simulink model "mf14_100"  (R2023b)
(part 2 of 10)

  u80/1 -> Sum158/2
  Sum123/1 -> Stick Input51/1, Controller51/1(Stick Input (in))
  Nz pilot calculation78/1(Pilot g force (g)) -> Pilot G force Scope78/1, Nz Pilot (g)84/1
  Dryden Wind Gust Models64/1(Wg) -> Gain220/1, Gain206/1  "wGust"
  Gain231/1 -> Sum174/1
  Sum177/1 -> Stick Input78/1, Controller78/1(Stick Input (in))
  Sum162/1 -> Stick Input80/1, Controller80/1(Stick Input (in))
  Pilot62/1 -> Sum145/1
  Sum113/1 -> Aircraft Dynamics Model52/3(Rotary Gust qGust (rad/sec))
  Controller77/1(Elevator Command (deg)) -> Actuator Model77/1
  Nz pilot calculation77/1(Pilot g force (g)) -> Pilot G force Scope77/1, Nz Pilot (g)83/1
  Controller70/1(Elevator Command (deg)) -> Actuator Model70/1
  Nz pilot calculation80/1(Pilot g force (g)) -> Pilot G force Scope80/1, Nz Pilot (g)86/1
  Sum104/1 -> Aircraft Dynamics Model96/3(Rotary Gust qGust (rad/sec))
  Gain237/1 -> alpha (rad)84/1, Angle of Attack78/1, Controller78/2(alpha (rad))
  Dryden Wind Gust Models78/2(Qg) -> Gain233/1  "qGust"
  Actuator Model81/1 -> Aircraft Dynamics Model81/1(Elevator Deflection d (deg))
  Dryden Wind Gust Models76/2(Qg) -> Gain267/1  "qGust"
  Gain221/1 -> alpha (rad)71/1, Angle of Attack64/1, Controller64/2(alpha (rad))
  Gain333/1 -> Sum106/2
  Dryden Wind Gust Models59/1(Wg) -> Gain351/1, Gain370/1  "wGust"
  Controller80/1(Elevator Command (deg)) -> Actuator Model80/1
  Gain367/1 -> alpha (rad)51/1, Angle of Attack51/1, Controller51/2(alpha (rad))
  Dryden Wind Gust Models87/1(Wg) -> Gain271/1, Gain310/1  "wGust"
  u56/1 -> Sum105/2
  Sum109/1 -> Stick Input98/1, Controller98/1(Stick Input (in))
  Aircraft Dynamics Model61/2(Pitch Rate q (rad/sec)) -> Nz pilot calculation61/2(q), Controller61/3(q (rad/sec))  "q"
  Dryden Wind Gust Models74/1(Wg) -> Gain238/1, Gain225/1  "wGust"
  Gain309/1 -> alpha (rad)91/1, Angle of Attack86/1, Controller86/2(alpha (rad))
  Nz pilot calculation99/1(Pilot g force (g)) -> Pilot G force Scope99/1, Nz Pilot (g)59/1
  Pilot91/1 -> Sum184/1
  Sum101/1 -> Stick Input50/1, Controller50/1(Stick Input (in))
  Sum138/1 -> Stick Input68/1, Controller68/1(Stick Input (in))
  Actuator Model97/1 -> Aircraft Dynamics Model97/1(Elevator Deflection d (deg))
  Sum157/1 -> Aircraft Dynamics Model74/3(Rotary Gust qGust (rad/sec))
  Controller62/1(Elevator Command (deg)) -> Actuator Model62/1
  Aircraft Dynamics Model75/1(Vertical Velocity w (ft/sec)) -> Gain265/1, Nz pilot calculation75/1(w)  "w"
  Gain287/1 -> Aircraft Dynamics Model93/2(Vertical Gust wGust (ft/sec))
  u91/1 -> Sum193/2
  Nz pilot calculation51/1(Pilot g force (g)) -> Pilot G force Scope51/1, Nz Pilot (g)51/1
  Sum187/1 -> Aircraft Dynamics Model93/3(Rotary Gust qGust (rad/sec))
  Aircraft Dynamics Model76/1(Vertical Velocity w (ft/sec)) -> Gain228/1, Nz pilot calculation76/1(w)  "w"
  u98/1 -> Sum188/2
  Sum199/1 -> Stick Input89/1, Controller89/1(Stick Input (in))
  Gain380/1 -> Sum135/2
  Gain259/1 -> alpha (rad)86/1, Angle of Attack80/1, Controller80/2(alpha (rad))
  Gain318/1 -> Sum108/2
  Dryden Wind Gust Models85/2(Qg) -> Gain270/1  "qGust"
  Gain248/1 -> Sum168/2
  Nz pilot calculation56/1(Pilot g force (g)) -> Pilot G force Scope56/1, Nz Pilot (g)64/1
  Sum128/1 -> Aircraft Dynamics Model54/3(Rotary Gust qGust (rad/sec))
  Dryden Wind Gust Models90/1(Wg) -> Gain297/1, Gain283/1  "wGust"
  Gain250/1 -> Aircraft Dynamics Model75/2(Vertical Gust wGust (ft/sec))
  Gain292/1 -> Sum190/2
  Gain308/1 -> Sum192/1
  Aircraft Dynamics Model85/2(Pitch Rate q (rad/sec)) -> Nz pilot calculation85/2(q), Controller85/3(q (rad/sec))  "q"
  Nz pilot calculation86/1(Pilot g force (g)) -> Pilot G force Scope86/1, Nz Pilot (g)91/1
  Gain307/1 -> alpha (rad)90/1, Angle of Attack85/1, Controller85/2(alpha (rad))
  Sum144/1 -> Stick Input71/1, Controller71/1(Stick Input (in))
  Controller92/1(Elevator Command (deg)) -> Actuator Model92/1
  Gain234/1 -> alpha (rad)83/1, Angle of Attack77/1, Controller77/2(alpha (rad))
  Sum179/1 -> Aircraft Dynamics Model85/3(Rotary Gust qGust (rad/sec))
  u90/1 -> Sum180/2
  Gain270/1 -> Sum179/2
  Gain364/1 -> Aircraft Dynamics Model58/2(Vertical Gust wGust (ft/sec))
  Pilot70/1 -> Sum142/1
  Pilot80/1 -> Sum162/1
  Sum135/1 -> Aircraft Dynamics Model63/3(Rotary Gust qGust (rad/sec))
  Actuator Model71/1 -> Aircraft Dynamics Model71/1(Elevator Deflection d (deg))
  Aircraft Dynamics Model92/2(Pitch Rate q (rad/sec)) -> Nz pilot calculation92/2(q), Controller92/3(q (rad/sec))  "q"
  Sum117/1 -> Aircraft Dynamics Model58/3(Rotary Gust qGust (rad/sec))
  Gain286/1 -> alpha (rad)97/1, Angle of Attack92/1, Controller92/2(alpha (rad))
  Gain360/1 -> Aircraft Dynamics Model53/2(Vertical Gust wGust (ft/sec))
  Gain219/1 -> alpha (rad)70/1, Angle of Attack63/1, Controller63/2(alpha (rad))
  Gain365/1 -> Sum117/2
  u97/1 -> Sum186/2
  Dryden Wind Gust Models86/1(Wg) -> Gain308/1, Gain294/1  "wGust"
  Gain304/1 -> Aircraft Dynamics Model92/2(Vertical Gust wGust (ft/sec))
  Controller79/1(Elevator Command (deg)) -> Actuator Model79/1
  u61/1 -> Sum127/2
  Aircraft Dynamics Model98/1(Vertical Velocity w (ft/sec)) -> Gain322/1, Nz pilot calculation98/1(w)  "w"
  Aircraft Dynamics Model79/2(Pitch Rate q (rad/sec)) -> Nz pilot calculation79/2(q), Controller79/3(q (rad/sec))  "q"
  Aircraft Dynamics Model90/1(Vertical Velocity w (ft/sec)) -> Gain300/1, Nz pilot calculation90/1(w)  "w"
  Aircraft Dynamics Model82/1(Vertical Velocity w (ft/sec)) -> Gain249/1, Nz pilot calculation82/1(w)  "w"
  Controller82/1(Elevator Command (deg)) -> Actuator Model82/1
  Sum196/1 -> Aircraft Dynamics Model88/3(Rotary Gust qGust (rad/sec))
  Actuator Model91/1 -> Aircraft Dynamics Model91/1(Elevator Deflection d (deg))
  u64/1 -> Sum133/2
  Aircraft Dynamics Model93/1(Vertical Velocity w (ft/sec)) -> Gain293/1, Nz pilot calculation93/1(w)  "w"
  Sum185/1 -> Aircraft Dynamics Model92/3(Rotary Gust qGust (rad/sec))
  Gain285/1 -> Sum185/1
  Gain335/1 -> Aircraft Dynamics Model52/2(Vertical Gust wGust (ft/sec))
  u69/1 -> Sum125/2
  Dryden Wind Gust Models84/1(Wg) -> Gain290/1, Gain257/1  "wGust"
  Dryden Wind Gust Models92/2(Qg) -> Gain305/1  "qGust"
  Nz pilot calculation90/1(Pilot g force (g)) -> Pilot G force Scope90/1, Nz Pilot (g)95/1
  u82/1 -> Sum173/2
  Nz pilot calculation92/1(Pilot g force (g)) -> Pilot G force Scope92/1, Nz Pilot (g)97/1
  Nz pilot calculation68/1(Pilot g force (g)) -> Pilot G force Scope68/1, Nz Pilot (g)75/1
  Sum111/1 -> Stick Input99/1, Controller99/1(Stick Input (in))
  Sum147/1 -> Stick Input72/1, Controller72/1(Stick Input (in))
  Dryden Wind Gust Models89/2(Qg) -> Gain277/1  "qGust"
  Dryden Wind Gust Models83/1(Wg) -> Gain251/1, Gain247/1  "wGust"
  Controller67/1(Elevator Command (deg)) -> Actuator Model67/1
  Controller98/1(Elevator Command (deg)) -> Actuator Model98/1
  Gain358/1 -> Sum124/2
  Dryden Wind Gust Models92/1(Wg) -> Gain285/1, Gain304/1  "wGust"
  Pilot86/1 -> Sum193/1
  Actuator Model94/1 -> Aircraft Dynamics Model94/1(Elevator Deflection d (deg))
  Dryden Wind Gust Models93/1(Wg) -> Gain289/1, Gain287/1  "wGust"
  Aircraft Dynamics Model63/2(Pitch Rate q (rad/sec)) -> Nz pilot calculation63/2(q), Controller63/3(q (rad/sec))  "q"
  Dryden Wind Gust Models88/1(Wg) -> Gain275/1, Gain273/1  "wGust"
  Aircraft Dynamics Model93/2(Pitch Rate q (rad/sec)) -> Nz pilot calculation93/2(q), Controller93/3(q (rad/sec))  "q"
  Gain279/1 -> alpha (rad)53/1, Angle of Attack73/1, Controller73/2(alpha (rad))
  Gain351/1 -> Sum119/1
  Aircraft Dynamics Model94/1(Vertical Velocity w (ft/sec)) -> Gain296/1, Nz pilot calculation94/1(w)  "w"
  Gain269/1 -> Aircraft Dynamics Model85/2(Vertical Gust wGust (ft/sec))
  Pilot93/1 -> Sum188/1
  Sum154/1 -> Aircraft Dynamics Model67/3(Rotary Gust qGust (rad/sec))
  Pilot88/1 -> Sum197/1
  Actuator Model93/1 -> Aircraft Dynamics Model93/1(Elevator Deflection d (deg))
  Dryden Wind Gust Models94/1(Wg) -> Gain295/1, Gain291/1  "wGust"
  Nz pilot calculation59/1(Pilot g force (g)) -> Pilot G force Scope59/1, Nz Pilot (g)67/1
  Aircraft Dynamics Model94/2(Pitch Rate q (rad/sec)) -> Nz pilot calculation94/2(q), Controller94/3(q (rad/sec))  "q"
  Pilot92/1 -> Sum186/1
  Aircraft Dynamics Model72/1(Vertical Velocity w (ft/sec)) -> Gain208/1, Nz pilot calculation72/1(w)  "w"
  Gain373/1 -> alpha (rad)60/1, Angle of Attack52/1, Controller52/2(alpha (rad))
  Gain302/1 -> Sum183/1
  Controller90/1(Elevator Command (deg)) -> Actuator Model90/1
  Nz pilot calculation76/1(Pilot g force (g)) -> Pilot G force Scope76/1, Nz Pilot (g)82/1
  Dryden Wind Gust Models88/2(Qg) -> Gain274/1  "qGust"
  Actuator Model72/1 -> Aircraft Dynamics Model72/1(Elevator Deflection d (deg))
  Aircraft Dynamics Model56/2(Pitch Rate q (rad/sec)) -> Nz pilot calculation56/2(q), Controller56/3(q (rad/sec))  "q"
  Sum164/1 -> Stick Input81/1, Controller81/1(Stick Input (in))
  Aircraft Dynamics Model52/2(Pitch Rate q (rad/sec)) -> Nz pilot calculation52/2(q), Controller52/3(q (rad/sec))  "q"
  Actuator Model75/1 -> Aircraft Dynamics Model75/1(Elevator Deflection d (deg))
  Gain346/1 -> Sum132/1
  Dryden Wind Gust Models98/1(Wg) -> Gain319/1, Gain317/1  "wGust"
  Actuator Model85/1 -> Aircraft Dynamics Model85/1(Elevator Deflection d (deg))
  Gain339/1 -> Aircraft Dynamics Model55/2(Vertical Gust wGust (ft/sec))
  Aircraft Dynamics Model58/1(Vertical Velocity w (ft/sec)) -> Gain369/1, Nz pilot calculation58/1(w)  "w"
  Sum126/1 -> Aircraft Dynamics Model53/3(Rotary Gust qGust (rad/sec))
  Gain228/1 -> alpha (rad)82/1, Angle of Attack76/1, Controller76/2(alpha (rad))
  Sum190/1 -> Aircraft Dynamics Model94/3(Rotary Gust qGust (rad/sec))
  Dryden Wind Gust Models97/2(Qg) -> Gain333/1  "qGust"
  Dryden Wind Gust Models80/1(Wg) -> Gain258/1, Gain254/1  "wGust"
  Aircraft Dynamics Model73/1(Vertical Velocity w (ft/sec)) -> Gain279/1, Nz pilot calculation73/1(w)  "w"
  Gain213/1 -> alpha (rad)52/1, Angle of Attack62/1, Controller62/2(alpha (rad))
  Gain344/1 -> alpha (rad)63/1, Angle of Attack55/1, Controller55/2(alpha (rad))
  Dryden Wind Gust Models60/1(Wg) -> Gain355/1, Gain353/1  "wGust"
  Sum130/1 -> Aircraft Dynamics Model55/3(Rotary Gust qGust (rad/sec))
  Dryden Wind Gust Models99/2(Qg) -> Gain321/1  "qGust"
  Gain355/1 -> Sum121/1
  Sum132/1 -> Aircraft Dynamics Model56/3(Rotary Gust qGust (rad/sec))
  Actuator Model55/1 -> Aircraft Dynamics Model55/1(Elevator Deflection d (deg))
  Gain293/1 -> alpha (rad)98/1, Angle of Attack93/1, Controller93/2(alpha (rad))
  Gain249/1 -> alpha (rad)88/1, Angle of Attack82/1, Controller82/2(alpha (rad))
  Sum102/1 -> Aircraft Dynamics Model95/3(Rotary Gust qGust (rad/sec))
  Gain256/1 -> alpha (rad)85/1, Angle of Attack79/1, Controller79/2(alpha (rad))
  Nz pilot calculation57/1(Pilot g force (g)) -> Pilot G force Scope57/1, Nz Pilot (g)65/1
  Dryden Wind Gust Models55/2(Qg) -> Gain340/1  "qGust"
  Controller55/1(Elevator Command (deg)) -> Actuator Model55/1
  u52/1 -> Sum145/2
  Nz pilot calculation93/1(Pilot g force (g)) -> Pilot G force Scope93/1, Nz Pilot (g)98/1
  Aircraft Dynamics Model55/2(Pitch Rate q (rad/sec)) -> Nz pilot calculation55/2(q), Controller55/3(q (rad/sec))  "q"
  Dryden Wind Gust Models77/1(Wg) -> Gain231/1, Gain229/1  "wGust"
  Sum120/1 -> Stick Input59/1, Controller59/1(Stick Input (in))
  Dryden Wind Gust Models55/1(Wg) -> Gain341/1, Gain339/1  "wGust"
  Pilot99/1 -> Sum111/1
  Aircraft Dynamics Model75/2(Pitch Rate q (rad/sec)) -> Nz pilot calculation75/2(q), Controller75/3(q (rad/sec))  "q"
  Sum167/1 -> Stick Input73/1, Controller73/1(Stick Input (in))
  Controller73/1(Elevator Command (deg)) -> Actuator Model73/1
  Aircraft Dynamics Model56/1(Vertical Velocity w (ft/sec)) -> Gain347/1, Nz pilot calculation56/1(w)  "w"
  Controller56/1(Elevator Command (deg)) -> Actuator Model56/1
  Gain327/1 -> Aircraft Dynamics Model96/2(Vertical Gust wGust (ft/sec))
  Dryden Wind Gust Models82/2(Qg) -> Gain244/1  "qGust"
  Gain289/1 -> Sum187/1
  Sum131/1 -> Stick Input55/1, Controller55/1(Stick Input (in))
  Actuator Model56/1 -> Aircraft Dynamics Model56/1(Elevator Deflection d (deg))
  Aircraft Dynamics Model57/1(Vertical Velocity w (ft/sec)) -> Gain366/1, Nz pilot calculation57/1(w)  "w"
  Dryden Wind Gust Models67/2(Qg) -> Gain387/1  "qGust"
  Actuator Model60/1 -> Aircraft Dynamics Model60/1(Elevator Deflection d (deg))
  Dryden Wind Gust Models96/2(Qg) -> Gain328/1  "qGust"
  Pilot56/1 -> Sum133/1
  Gain245/1 -> Sum165/1
  Aircraft Dynamics Model51/1(Vertical Velocity w (ft/sec)) -> Gain367/1, Nz pilot calculation51/1(w)  "w"
  Sum186/1 -> Stick Input92/1, Controller92/1(Stick Input (in))
  Sum166/1 -> Stick Input82/1, Controller82/1(Stick Input (in))
  Dryden Wind Gust Models79/2(Qg) -> Gain240/1  "qGust"
  Gain306/1 -> Sum192/2
  Nz pilot calculation89/1(Pilot g force (g)) -> Pilot G force Scope89/1, Nz Pilot (g)94/1
  Aircraft Dynamics Model59/2(Pitch Rate q (rad/sec)) -> Nz pilot calculation59/2(q), Controller59/3(q (rad/sec))  "q"
  Pilot52/1 -> Sum114/1
